simulink model "testsim"  (R2018b)
settings: Solver=ode4  StartTime=0.0  StopTime=10  FixedStep=0.001  RelTol=1e-3  EnableMultiTasking=on
libraries: simulink x1
settings Model: ExtModeTrigMode=oneshot  ExtModeArmWhenConnect=off  Creator=hp  LastModifiedBy=Administrator
settings SolverCC: AlgebraicLoopSolver=LineSearch
settings DataIOCC: SaveFormat=Array  SignalLoggingSaveFormat=ModelDataLogs  SignalLoggingName=sigsOut
settings OptimizationCC: BooleanDataType=off  ExpressionDepthLimit=2147483647  InitFltsAndDblsToZero=on  LifeSpan=inf
settings DebuggingCC: SaveWithParameterizedLinksMsg=none  UnderspecifiedInitializationDetection=Classic  MergeDetectMultiDrivingBlocksExec=none  SignalResolutionControl=TryResolveAllWithWarning  MultiTaskDSMMsg=warning  MultiTaskCondExecSysMsg=none  FcnCallInpInsideContextMsg=warning  StateNameClashWarn=warning  SFUnexpectedBacktrackingDiag=warning  SFNoUnconditionalDefaultTransitionDiag=warning  SFExecutionAtInitializationDiag=none
settings HardwareCC: ProdBitPerPointer=32  ProdBitPerSizeT=32  ProdBitPerPtrDiffT=32  ProdLargestAtomicFloat=None  ProdIntDivRoundTo=Undefined  ProdEndianess=Unspecified  ProdWordSize=32  ProdHWDeviceType=32-bit Generic  TargetUnknown=on
settings ModelReferenceCC: PropagateSignalLabelsOutOfModel=off
settings SFSimCC: SimUseLocalCustomCode=off
settings RTWCC: RTWUseLocalCustomCode=off
settings CodeAppCC: StateflowObjectComments=on
settings GRTTargetCC: TargetFcnLib=ansi_tfl_tmw.mat  TargetLangStandard=C89/C90 (ANSI)  GeneratePreprocessorConditionals=Disable all  CombineOutputUpdateFcns=off  GRTInterface=on
settings ConfigComp: CovMetricSettings=dw  CovHtmlReporting=on  CovSaveCumulativeToWorkspaceVar=on  CovSaveSingleToWorkspaceVar=on  CovExternalEMLEnable=off

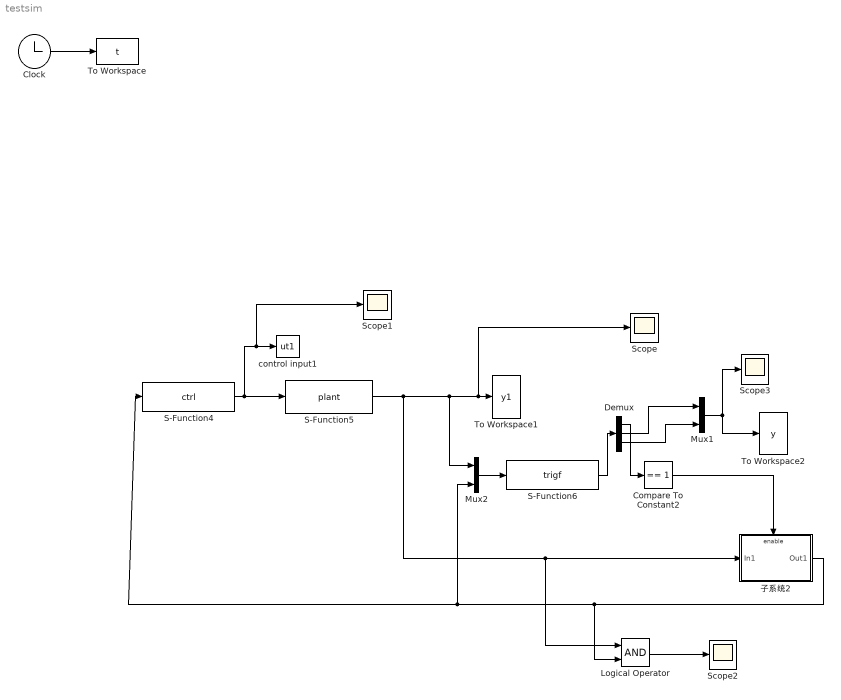
== system testsim ==
  Clock : Clock
  Compare To Constant2 : simulink/Logic and Bit Operations/Compare To Constant  relop===  const=1  OutDataTypeStr=boolean
  Demux : Demux  Outputs=3
  Logical Operator : Logic  AllPortsSameDT=off  OutDataTypeStr=boolean
  Mux1 : Mux  Inputs=2
  Mux2 : Mux  Inputs=2
  S-Function4 : S-Function  FunctionName=ctrl  SFunctionDeploymentMode=off  EnableBusSupport=off
  S-Function5 : S-Function  FunctionName=plant  SFunctionDeploymentMode=off  EnableBusSupport=off
  S-Function6 : S-Function  FunctionName=trigf  SFunctionDeploymentMode=off  EnableBusSupport=off
  Scope{,1..3} (4 alike) : Scope
  To Workspace : ToWorkspace  VariableName=t  SampleTime=-1
  To Workspace1 : ToWorkspace  VariableName=y1  SampleTime=-1
  To Workspace2 : ToWorkspace  VariableName=y  SampleTime=-1
  control input1 : ToWorkspace  VariableName=ut1  SampleTime=-1
  子系统2 : Subsystem  TreatAsAtomicUnit=on
  wires:
  Clock/1 -> To Workspace/1
  Mux2/1 -> S-Function6/1
  S-Function5/1 -> Logical Operator/1, 子系统2/1(In1), Scope/1, To Workspace1/1, Mux2/1
  S-Function4/1 -> Scope1/1, control input1/1, S-Function5/1
  Compare To Constant2/1 -> 子系统2/Enable
  子系统2/1(Out1) -> Logical Operator/2, S-Function4/1, Mux2/2
  Logical Operator/1 -> Scope2/1
  S-Function6/1 -> Demux/1
  Demux/1 -> Compare To Constant2/1
  Demux/3 -> Mux1/2
  Demux/2 -> Mux1/1
  Mux1/1 -> To Workspace2/1, Scope3/1

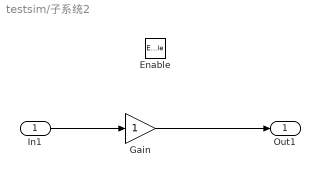
== system testsim/子系统2 ==
  In1 : Inport
  Enable : EnablePort
  Gain : Gain
  Out1 : Outport  VectorParamsAs1DForOutWhenUnconnected=on
  wires:
  In1/1 -> Gain/1
  Gain/1 -> Out1/1
